simulink model "testemplanner_cs"  (R2023a)
settings: Solver=ode5  StartTime=0.0  StopTime=70  FixedStep=1/1000  RelTol=1e-3
PreLoadFcn:
  | mbxruntime.callbacks.PreLoadFcn(bdroot);
PostLoadFcn:
  | mbxruntime.callbacks.PostLoadFcn(bdroot);
InitFcn:
  | mbxruntime.callbacks.InitFcn(bdroot);
StartFcn:
  | mbxruntime.callbacks.StartFcn(bdroot);
StopFcn:
  | mbxruntime.callbacks.StopFcn(bdroot);
model workspace (MAT data in the model file):
  mbox_table : object (value not decoded)
  model_closed = 0
  sim_status = 0
values from neighbouring files (symbols this model uses):
  c_factor = 43.75    [emplanner_init.m]
  cf = -175016    [emplanner_init.m]
  cr = -130634    [emplanner_init.m]
  global_path_x = [-4.4795 -3.48011774493 -2.48199463442 -1.48514775065 -0.489582877207 0.504698358082 1.49769585569 2.48941007764 3.47984169183 4.46899144113 5.45686009523 6.44344843293 ... (3001 elements, 3001x1)]    [global_path.mat]
  global_path_y = [6.0531 6.0531 6.0531 6.0531 6.0531 6.0531 6.0531 6.0531 6.0531 6.0531 6.0531 6.0531 ... (3001 elements, 3001x1)]    [global_path.mat]
  KD_PID_distance = 0.0    (= 0)    [emplanner_init.m]
  KD_PID_speed = 0    [emplanner_init.m]
  KI_PID_distance = 0.0    (= 0)    [emplanner_init.m]
  KI_PID_speed = 0    [emplanner_init.m]
  KP_PID_distance = 0.5    [emplanner_init.m]
  KP_PID_speed = 1.8    [emplanner_init.m]
  la = 1.265    [emplanner_init.m]
  lb = 2.947-1.265    (= 1.682)    [emplanner_init.m]
  LQR_K1 = k(:,1)'    [emplanner_init.m]
  LQR_K2 = k(:,2)'    [emplanner_init.m]
  LQR_K3 = k(:,3)'    [emplanner_init.m]
  LQR_K4 = k(:,4)'    [emplanner_init.m]
  m = 2020    [emplanner_init.m]
  rack_displacement = [-39.14 , -37.2 , -35.29 , -33.43 , -31.6 , -29.81 , -28.06 , -26.34 , -24.66 ,      -23.01 , -21.38 , -19.79 , -18.23 , -16.69 , -15.18 , -13.7 , -12.23 , -10.8 , -9.38 , -7.98 ,     -6.61 , -5.25 , -3.91 , -2.59 , -1.29 , 0 , 1.27 , 2.54 , 3.78 , 5.02 , 6.24 , 7.46 , 8.66 ,      9.86 , 11.05 , 12.24 , 13.41 , 14.59 , 15.76 , 16.92 , 18.09 , 19.25 , 20.42 , 21.59 , 22.76 ,      23.93 , 25.11 , 26 ...(+26 chars)    [emplanner_init.m]
  right_wheel_ground = [-70 ,-67.2 , -64.4 , -61.6 , -58.8 , -56 , -53.2 , -50.4 , -47.6 , -44.8 , -42 ,      -39.2 , -36.4 , -33.6 , -30.8 , -28 , -25.2 , -22.4 , -19.6 , -16.8 , -14 , -11.2 , -8.4 , -5.6 ,      -2.8 , 0 , 2.8 , 5.6 , 8.4 , 11.2 , 14 , 16.8 , 19.6 , 22.4 , 25.2 , 28 , 30.8 , 33.6 , 36.4 ,      39.2 , 42 , 44.8 , 47.6 , 50.4 , 53.2 , 56 , 58.8 , 61.6 , 64.4 , 67.2 , 70 ]    [emplanner_init.m]
  vx_break_point = zeros(1,5000)    [emplanner_init.m]
undefined symbols (not defined in the file or in its folder): aubr, DiscIntNeverNeededParam, tablebr, vubr, warningInitialVelocity, x0
libraries: PreScanSimulinkLibrary x19, simulink x19, simulink_extras x6, Solver_SF x1
(part 9 of 10)

== matlab function testemplanner_cs/Audi_A8_Sedan_1/decision&planning module/EM Planner/Dynamic Programming ==
  data: dp_path_s output; dp_path_l output; planning_start_s input; planning_start_l input; planning_start_dl input; planning_start_ddl input; obs_s_set input; obs_l_set input; row input; col input; sample_s input; sample_l input; w_dl_smooth_cost input; w_ddl_smooth_cost input; w_dddl_smooth_cost input; w_reference_cost input; w_collision_cost input
function [dp_path_s, dp_path_l] = fcn(planning_start_s, planning_start_l, planning_start_dl, planning_start_ddl, obs_s_set,...
    obs_l_set, row, col, sample_s, sample_l, w_dl_smooth_cost, w_ddl_smooth_cost, w_dddl_smooth_cost, w_reference_cost, w_collision_cost)

%该函数是动态规划（决策算法）的主函数
%要写的太多了，想起什么写什么吧

%node_cost(i,j)为起点到当前节点的最小代价
%每一列中有一个最小的数，代表起点到该列的最小代价
%最后一列的最小数即为起点到最后一列的最小代价，即为我们需要的粗解

%初始化
node_cost = ones(row, col)*inf;
point_s = zeros(row,col);
point_l = zeros(row, col);
point_dl = zeros(row, col);
point_ddl = zeros(row, col);

%下面会计算起点到第一列的最小代价
for i = 1:row
    point_s(i, 1) = planning_start_s+sample_s;
    %对于某奇数行的点阵，例如row=3,point_l(11)=1*sample_l,point_l(31)=-1*sample_l
    point_l(i, 1) = ((row+1)/2-i)*sample_l;
    %用五次多项式连接起点到刚刚生成的点
    %五次多项式有六个边界条件
    start_l = planning_start_l;
    start_dl = planning_start_dl;
    start_ddl = 0;
    end_l = ((row+1)/2-i)*sample_l;
    end_dl = 0;
    end_ddl = 0;
    start_s = planning_start_s;
    end_s = planning_start_s+sample_s;
    %下面定义根据起点中点的六个边界条件计算五次多项式
    cofficient = CalcPathFiveCoff(start_s, end_s, start_l, start_dl, start_ddl, end_l, end_dl, end_ddl);

    %已经将起点和第一列的第一个点用五次多项式连接起来，将六个系数提取出来
    a0 = cofficient(1);
    a1 = cofficient(2);
    a2 = cofficient(3);
    a3 = cofficient(4);
    a4 = cofficient(5);
    a5 = cofficient(6);

    %在曲线上均匀提取十个采样点
    sample_point_s = zeros(10,1);
    sample_point_l = zeros(10,1);
    sample_point_dl = zeros(10,1);
    sample_point_ddl = zeros(10,1);
    sample_point_dddl = zeros(10,1);
    for j = 1:10
        sample_point_s(j) = start_s+j*sample_s/10; %（第一个）采样点的s
    end

    %五次多项式为：a0+a1*s+a2*s^2+a3*s^3+a4*s^4+a5*s^5,根据采样点s计算l,dl,ddl,dddl
    sample_point_l = a0+a1*sample_point_s+a2*sample_point_s.^2+a3*sample_point_s.^3+a4*sample_point_s.^4+...
        a5*sample_point_s.^5;
    sample_point_dl = a1+2*a2*sample_point_s+3*a3*sample_point_s.^2+4*a4*sample_point_s.^3+5*a5*sample_point_s.^4;
    sample_point_ddl = 2*a2+6*a3*sample_point_s+12*a4*sample_point_s.^2+20*a5*sample_point_s.^3;
    sample_point_dddl = 6*a3+24*a4*sample_point_s+60*a5*sample_point_s.^2;
    
    %计算平滑代价、参考线距离代价
    smooth_cost = w_dl_smooth_cost*(sample_point_dl'*sample_point_dl)+w_ddl_smooth_cost*(sample_point_ddl'*sample_point_ddl)...
        +w_dddl_smooth_cost*(sample_point_dddl'*sample_point_dddl);
    reference_cost = w_reference_cost*(sample_point_l'*sample_point_l);

    %定义障碍物代价函数,遍历每个障碍物计算代价做累加
    collision_cost = 0;
    for k = 1:length(obs_s_set)
        if isnan(obs_s_set(k))
            break;
        end
        collision_cost_once = CalcCollCost(sample_point_s, sample_point_l, obs_s_set(k), obs_l_set(k), w_collision_cost);
        collision_cost = collision_cost+collision_cost_once; 
    end

    %计算第一列每个点到起点的node_cost
    node_cost(i, 1) = smooth_cost+reference_cost+collision_cost;

end

%下面将计算从第二列开始每一个点的node_cost
%定义pre_node_index，用来记录当前点的最优路径下，上一个点所对应的行号（列号为当前点-1，无需记录）
%例如有如下点阵,最优路径为（33）<（22）<(11)
%...
%...
%...
%则pre_node_index(33)=2,pre_node_index(22)=1,pre_node_index(11)=0(行数0表示起点)

%初始化pre_node_index矩阵，其值均设为0
pre_node_index = zeros(row, col);

%下面是动态规划的主函数(从第二列开始)
for j = 2:col
    for i = 1:row
        %例如node_cost(1,j)=node_cost(i,j-1)+neighbor_cost(i,j-1)>(1,j)
        %下面要写遍历算法，记录下第二列每个点的node_cost（遍历的是第一列每个点的代价）及pre_node_index
        current_point_s = planning_start_s+j*sample_s;
        current_point_l = ((row+1)/2-i)*sample_l;
        for k = 1:row
            %调用计算相邻点代价的函数
            start_point_s = planning_start_s+(j-1)*sample_s;
            start_point_l = ((row+1)/2-k)*sample_l;
            neighbor_cost = CalcNeighborCost(start_point_s, start_point_l, w_dl_smooth_cost...
            , w_ddl_smooth_cost, w_dddl_smooth_cost, sample_s, obs_s_set, current_point_s, ...
            current_point_l);
            temp_node_cost = node_cost(k, j-1)+neighbor_cost;
            if temp_node_cost < node_cost(i, j)
                node_cost(i, j) = temp_node_cost;
                pre_node_index(i, j) = k;
            end

        end
    end
end

%到这里就写完了动态规划的大部分内容，可以遍历最后一列得到最小代价，以及此路径对应的上一列的行数
%反向递推到第一列就获得了动态规划的结果（粗解）

%row_line（i)为粗解的第i列所对应的行号
row_line = zeros(col, 1);
min_node_cost = inf;

for i = 1:row
    if node_cost(i, col) < min_node_cost
        min_node_cost = node_cost(i, col);
        row_line(col) = i;
    end
end

%映射最优点的pre_node_index,也就是上一列的行号
for j = col-1:-1:1
    row_line(j) = pre_node_index(row_line(j+1), j+1);
end

%将输出初始化，由于事先不知道横纵向的采样数，因此要做缓冲
dp_path_s = ones(15, 1)*-1;
dp_path_l = ones(15, 1)*-1;
for i = 1:col
    dp_path_s(i) = planning_start_s+i*sample_s;
    dp_path_l(i) = ((row+1)/2-row_line(i))*sample_l;
end

%这里定义计算临近点代价的函数，与第一列到起点代价的计算很接近，注意起始点dl,ddl不同...
    function neighbor_cost = CalcNeighborCost(start_point_s, start_point_l, w_dl_smooth_cost...
            , w_ddl_smooth_cost, w_dddl_smooth_cost, sample_s, obs_s_set, current_point_s, ...
            current_point_l)

        %用五次多项式连接起点到刚刚生成的点
        %五次多项式有六个边界条件
        start_l = start_point_l;
        start_dl = 0;
        start_ddl = 0;
        end_l = current_point_l;
        end_dl = 0;
        end_ddl = 0;
        start_s = start_point_s;
        end_s = current_point_s;
        %下面定义根据起点中点的六个边界条件计算五次多项式
        cofficient = CalcPathFiveCoff(start_s, end_s, start_l, start_dl, start_ddl, end_l, end_dl, end_ddl);
    
        %已经将起点和第一列的第一个点用五次多项式连接起来，将六个系数提取出来
        a0 = cofficient(1);
        a1 = cofficient(2);
        a2 = cofficient(3);
        a3 = cofficient(4);
        a4 = cofficient(5);
        a5 = cofficient(6);
    
        %在曲线上均匀提取十个采样点
        sample_point_s = zeros(10,1);
        sample_point_l = zeros(10,1);
        sample_point_dl = zeros(10,1);
        sample_point_ddl = zeros(10,1);
        sample_point_dddl = zeros(10,1);
        for m = 1:10
            sample_point_s(m) = start_s+m*sample_s/10; %（第一个）采样点的s
        end
    
        %五次多项式为：a0+a1*s+a2*s^2+a3*s^3+a4*s^4+a5*s^5,根据采样点s计算l,dl,ddl,dddl
        sample_point_l = a0+a1*sample_point_s+a2*sample_point_s.^2+a3*sample_point_s.^3+a4*sample_point_s.^4+...
            a5*sample_point_s.^5;
        sample_point_dl = a1+2*a2*sample_point_s+3*a3*sample_point_s.^2+4*a4*sample_point_s.^3+5*a5*sample_point_s.^4;
        sample_point_ddl = 2*a2+6*a3*sample_point_s+12*a4*sample_point_s.^2+20*a5*sample_point_s.^3;
        sample_point_dddl = 6*a3+24*a4*sample_point_s+60*a5*sample_point_s.^2;
        
        %计算平滑代价、参考线距离代价
        smooth_cost = w_dl_smooth_cost*(sample_point_dl'*sample_point_dl)+w_ddl_smooth_cost*(sample_point_ddl'*sample_point_ddl)...
            +w_dddl_smooth_cost*(sample_point_dddl'*sample_point_dddl);
        reference_cost = w_reference_cost*(sample_point_l'*sample_point_l);
    
        %定义障碍物代价函数,遍历每个障碍物计算代价做累加
        collision_cost = 0;
        for n = 1:length(obs_s_set)
            if isnan(obs_s_set(n))
                break;
            end
            collision_cost_once = CalcCollCost(sample_point_s, sample_point_l, obs_s_set(n), obs_l_set(n), w_collision_cost);
            collision_cost = collision_cost+collision_cost_once; 
        end
    
        %计算相邻两点的neighbor_cost
        neighbor_cost = smooth_cost+reference_cost+collision_cost;

    end

%在这里定义碰撞代价函数
    function collision_cost = CalcCollCost(sample_point_s, sample_point_l, obs_s, obs_l, w_collision_cost)

        collision_cost = 0; 
        %我们认为障碍物与自车距离大于4米时无代价，3<距离<4时代价为1000/square_distance,距离<3时代价为w_collision_cost
        %其中square_distance为ds^2+dl^2,也就是距离的平方
        ds = (obs_s*ones(10,1)-sample_point_s);
        dl = (obs_l*ones(10,1)-sample_point_l);
        square_distance = ds.^2+dl.^2;
        for q = 1:length(square_distance)
            if square_distance(q) > 9 && square_distance(q) < 16
                collision_cost = collision_cost+1000/square_distance(q);
            elseif square_distance(q) < 9
                collision_cost = collision_cost+w_collision_cost;        
            end
        end
    end

%在这里定义计算五次多项式的函数
function Path_Five_Coff = CalcPathFiveCoff(start_s, end_s, start_l, start_dl, start_ddl, end_l, end_dl, end_ddl)
    %l = a0+a1*s+a2*s^2+a3*s^3+a4*s^4+a5*s^5
    %dl = a1+2*a2*s+3*a3*s^2+4*a4*s^3+5*a5*s^4
    %ddl = 2*a2+6*a3*s+12*a4*s^2+20*a5*s^3
    
    A = [1, start_s, start_s^2, start_s^3, start_s^4, start_s^5;
         0, 1, 2*start_s, 3*start_s^2, 4*start_s^3, 5*start_s^4;
         0, 0, 2, 6*start_s, 12*start_s^2, 20*start_s^3;
         1, end_s, end_s^2, end_s^3, end_s^4, end_s^5;
         0, 1, 2*end_s, 3*end_s^2, 4*end_s^3, 5*end_s^4;
         0, 0, 2, 6*end_s, 12*end_s^2, 20*end_s^3];

    B = [start_l;
         start_dl;
         start_ddl;
         end_l;
         end_dl;
         end_ddl];

    Path_Five_Coff = A\B;
end
end

== matlab function testemplanner_cs/Audi_A8_Sedan_1/decision&planning module/EM Planner/MATLAB Function ==
  data: dp_path_s_init input; dp_path_s_final output; dp_path_l_init input; plan_start_s input; plan_start_l input; plan_start_dl input; plan_start_ddl input; dp_path_l_final output; dp_path_dl_final output; dp_path_ddl_final output
function [dp_path_s_final, dp_path_l_final, dp_path_dl_final, dp_path_ddl_final] = fcn(dp_path_s_init, dp_path_l_init, plan_start_s, plan_start_l...
    , plan_start_dl, plan_start_ddl)

%dp_path_x_init中s方向每隔10m采样一个点，并不是一条密集连续的轨迹，要对轨迹增密
%我们并不知道s方向的采样间隔是多少（可能是10，12，15...），但传感器能探测到的范围大概为60m
%假设ds=1，即每隔1m采样一个点，设置最终轨迹的大小为60，即最多存储60个点（设置缓冲）

ds = 1;
dp_path_s_final = ones(60, 1)*nan;
dp_path_l_final = ones(60, 1)*nan;
dp_path_dl_final = ones(60, 1)*nan;
dp_path_ddl_final = ones(60, 1)*nan;

%设置动态数组用来存储采样点
l_temp = [];
dl_temp = [];
ddl_temp = [];

%设置五次多项式起点
start_s = plan_start_s;
start_l = plan_start_l;
start_dl = plan_start_dl;
start_ddl = plan_start_ddl;

for i = 1:length(dp_path_s_init)
    
    %声明一个动态数组存放采样点的s
    s_cur = [];

    if dp_path_s_init(i) == -1
        break;
    end
    
    %设置内层循环，终点是final_path_s_init(i)
    for j = 1:10000
        s_node = start_s+(j-1)*ds;
        if s_node < dp_path_s_init(i)
            s_cur = [s_cur, s_node];
        else
            break;
        end
    end

    %设置五次多项式终点
    end_s = dp_path_s_init(i);
    end_l = dp_path_l_init(i);
    end_dl = 0;
    end_ddl = 0;
    
    %调用五次多项式函数求解s_cur所对应的l
    Coff = CalcPathFiveCoff(start_s, end_s, start_l, start_dl, start_ddl, end_l, end_dl, end_ddl);
    a0 = Coff(1);
    a1 = Coff(2);
    a2 = Coff(3);
    a3 = Coff(4);
    a4 = Coff(5);
    a5 = Coff(6);
    l = a0*ones(1, length(s_cur))+a1*s_cur+a2*s_cur.^2+a3*s_cur.^3+a4*s_cur.^4+a5*s_cur.^5;
    dl = a1*ones(1, length(s_cur))+2*a2*s_cur+3*a3*s_cur.^2+4*a4*s_cur.^3+5*a5*s_cur.^4;
    ddl = 2*a2*ones(1, length(s_cur))+6*a3*s_cur+12*a4*s_cur.^2+20*a5*s_cur.^3;
    l_temp = [l_temp, l];
    dl_temp = [dl_temp, dl];
    ddl_temp = [ddl_temp, ddl];

    %给s,lfinal赋值，注意l,dl,ddl是扩展的，s_cur是一次性的，每次循环最后要清零
    for k = 1:length(l_temp)
        if k == 61
            break;
        end
        dp_path_s_final(k) = plan_start_s+(k-1)*ds;
        dp_path_l_final(k) = l_temp(k);
        dp_path_dl_final(k) = dl_temp(k);
        dp_path_ddl_final(k) = ddl_temp(k);
    end
 
    %为下一次循环赋值
    start_s = end_s;
    start_l = end_l;
    start_dl = end_dl;
    start_ddl = end_ddl;
   
end

end

%在这里定义计算五次多项式的函数
function Path_Five_Coff = CalcPathFiveCoff(start_s, end_s, start_l, start_dl, start_ddl, end_l, end_dl, end_ddl)
    %l = a0+a1*s+a2*s^2+a3*s^3+a4*s^4+a5*s^5
    %dl = a1+2*a2*s+3*a3*s^2+4*a4*s^3+5*a5*s^4
    %ddl = 2*a2+6*a3*s+12*a4*s^2+20*a5*s^3
    
    A = [1, start_s, start_s^2, start_s^3, start_s^4, start_s^5;
         0, 1, 2*start_s, 3*start_s^2, 4*start_s^3, 5*start_s^4;
         0, 0, 2, 6*start_s, 12*start_s^2, 20*start_s^3;
         1, end_s, end_s^2, end_s^3, end_s^4, end_s^5;
         0, 1, 2*end_s, 3*end_s^2, 4*end_s^3, 5*end_s^4;
         0, 0, 2, 6*end_s, 12*end_s^2, 20*end_s^3];

    B = [start_l;
         start_dl;
         start_ddl;
         end_l;
         end_dl;
         end_ddl];

    Path_Five_Coff = A\B;
end

== matlab function testemplanner_cs/Audi_A8_Sedan_1/decision&planning module/EM Planner/Frenet2Cartesian ==
  data: s_set input; l_set input; dl_set input; ddl_set input; frenet_x input; frenet_y input; frenet_heading input; frenet_kappa input; index2s input; x_point_set output; y_point_set output; heading_point_set output; kappa_point_set output
function [x_point_set, y_point_set, heading_point_set, kappa_point_set] = fcn(s_set, l_set, dl_set, ddl_set, frenet_x, ...
    frenet_y, frenet_heading, frenet_kappa, index2s)

%该函数的作用是把自然坐标系(s,l)下的粗解转换到笛卡尔坐标系（x,y）
%不确定有多少个点需要坐标转换，要做缓冲
%frenet转cartesian的步骤是：先找到待变换点在参考线上投影点的x,y，再计算待转换点的x,y

%在index2s上遍历得到匹配点编号，用匹配点求投影点的xy...

%这里可能有bug,因为s是点的投影的弧长，而不是点的匹配点的弧长，我认为找到在参考线上索引之后可以直接得到投影点的几何信息

x_point_set = ones(128, 1)*nan;
y_point_set = ones(128, 1)*nan;
heading_point_set = ones(128, 1)*nan;
kappa_point_set = ones(128, 1)*nan; 

for i = 1:length(s_set)
    if isnan(s_set(i))
        break;
    end
    %调用函数计算投影点
    [proj_point, proj_point_x, proj_point_y, proj_point_heading, proj_point_kappa] = CalcProjPoint(index2s, s_set(i), frenet_x, frenet_y, frenet_heading, frenet_kappa);
    %根据投影点的xy计算待转换点的xy
    proj_nor = [-sin(proj_point_heading); cos(proj_point_heading)];
    point = proj_point+proj_nor*l_set(i);
    x_point_set(i) = point(1);
    y_point_set(i) = point(2);
    heading_point_set(i) = atan(dl_set(i)/(1-proj_point_kappa*l_set(i)))+proj_point_heading;
    %近似认为kr'=0
    kappa_point_set(i) = ((ddl_set(i)+proj_point_kappa*dl_set(i)*tan(heading_point_set(i)-proj_point_heading))...
        *(cos(heading_point_set(i)-proj_point_heading)^2)/(1-proj_point_kappa*l_set(i))+proj_point_kappa)*cos(heading_point_set(i)-proj_point_heading)...
        /(1-proj_point_kappa*l_set(i));

end

end

%定义计算投影点的函数
function [proj_point, proj_point_x, proj_point_y, proj_point_heading, proj_point_kappa] = CalcProjPoint(index2s, s, frenet_x, frenet_y, frenet_heading, frenet_kappa)

%先遍历找到index2s上的匹配点
match_index = 1;
while index2s(match_index) < s
    match_index = match_index+1;
end
%提取数据（按照上述做法，匹配点一定在投影点之后，感觉有bug）
match_point = [frenet_x(match_index); frenet_y(match_index)];
match_point_heading = frenet_heading(match_index);
match_point_kappa = frenet_kappa(match_index);
ds = s-index2s(match_index);
match_tor = [cos(match_point_heading); sin(match_point_heading)];
proj_point = match_point+ds*match_tor;
proj_point_x = proj_point(1);
proj_point_y = proj_point(2);
proj_point_heading = match_point_heading+ds*match_point_kappa;
proj_point_kappa = match_point_kappa;
end

== matlab function testemplanner_cs/Audi_A8_Sedan_1/decision&planning module/referenceline provider/match&proj point search1 ==
  data: match_point_index_set output; proj_x_set output; proj_y_set output; proj_heading_set output; proj_kappa_set output; x_set input; y_set input; frenet_x_set input; frenet_y_set input; frenet_heading_set input; frenet_kapppa_set input
function [match_point_index_set, proj_x_set, proj_y_set, proj_heading_set, proj_kappa_set] = fcn(x_set, y_set, frenet_x_set, frenet_y_set, ...
    frenet_heading_set, frenet_kapppa_set)

%待投影点是一个集合（自车，障碍物），每一个点分别遍历寻找匹配点，再寻找投影点
%匹配点集合要保存下来，作为下次遍历开始的起点
%第一次遍历，没有任何提示，从frenet点集第一点开始遍历
%若不是第一次遍历，从上次保存的匹配点开始，注意方向
%待投影点-寻找匹配点-寻找投影点-投影点（x,y,heading,kappa），保存匹配点索引集合

%（待）投影点数量未知，设置缓冲，最多批量处理128个点,信息冗余用NAN（not a number）处理
n = 128;
match_point_index_set = ones(n,1)*nan;
proj_x_set = ones(n,1)*nan;
proj_y_set = ones(n,1)*nan;
proj_heading_set = ones(n,1)*nan;
proj_kappa_set = ones(n,1)*nan;

%两种情况：第一次遍历，非第一次遍历
%声明两个全局变量，第一个用来判断是否初次运行，第二个用来存储上次匹配点集合
persistent is_first_run
persistent pre_match_point_index_set

if isempty(is_first_run)
    is_first_run = 0;
    pre_match_point_index_set = ones(n,1)*nan;
    %遍历每一个点寻找匹配点
    start_search_index = 1;
    for i = 1:length(x_set)
        if isnan(x_set(i))
            break;
        end
        increase_count = 0;
        min_distant = inf;
        for j = start_search_index:length(frenet_x_set)
            distant = (x_set(i)-frenet_x_set(j))^2+(y_set(i)-frenet_y_set(j))^2;
            if distant < min_distant
                min_distant = distant;
                increase_count = 0;
                match_point_index_set(i) = j;
            else
                increase_count = increase_count+1;
            end
            %第一次遍历连续增加50次停止
            if increase_count > 50
                break;
            end
        end
        %通过匹配点计算投影点
        %计算匹配点的位矢及方向向量
        vector_match_point = [frenet_x_set(match_point_index_set(i));frenet_y_set(match_point_index_set(i))];
        vector_match_point_direction = [cos(frenet_heading_set(match_point_index_set(i)));sin(frenet_heading_set(match_point_index_set(i)))];
        vector_d = [x_set(i);y_set(i)]-vector_match_point;
        ds = vector_d'*vector_match_point_direction;
        vector_ds = ds*vector_match_point_direction;
        vector_proj_point = vector_match_point+vector_ds;
        %计算投影点的x,y,heading,kappa
        proj_x_set(i) = vector_proj_point(1);
        proj_y_set(i) = vector_proj_point(2);
        proj_heading_set(i) = frenet_heading_set(match_point_index_set(i))+frenet_kapppa_set(match_point_index_set(i))*ds;
        proj_kappa_set(i) = frenet_kapppa_set(match_point_index_set(i));
    end
    pre_match_point_index_set = match_point_index_set;
else
    %如果不是第一次遍历
    for i = 1:length(x_set)

        if isnan(x_set(i))
            break;
        end
        %下面这行代码有严重问题，需要投影的不仅是自车，还有障碍物
        %而第一次运行时传感器可能监测不到障碍物，即算法会跳过is first run分支执行else分支
        %此时pre_match_point_index_set中除了自车都是nan，所以需要修复
        start_search_index = pre_match_point_index_set(i);
        increase_count_limit = 5;

        if isnan(start_search_index)
            %从第一个点开始遍历，并需要遍历50次防止取到局部极小值
            increase_count_limit = 50;
            start_search_index = 1;
        end

        increase_count = 0;
        min_distant = inf;
        %判断遍历方向
        vector_pre_match_point = [frenet_x_set(start_search_index);frenet_y_set(start_search_index)];
        vector_pre_match_point_direction = [cos(frenet_heading_set(start_search_index));sin(frenet_heading_set(start_search_index))];
        flag = ([x_set(i);y_set(i)]-vector_pre_match_point)'*vector_pre_match_point_direction;
        

        %正向遍历
        if flag > 0.001
            for j = start_search_index:length(frenet_x_set)
                distant = (x_set(i)-frenet_x_set(j))^2+(y_set(i)-frenet_y_set(j))^2;
                if distant < min_distant
                    min_distant = distant;
                    increase_count = 0;
                    match_point_index_set(i) = j;
                else
                    increase_count = increase_count+1;
                end
                %连续增加5次停止
                if increase_count > increase_count_limit
                    break;
                end
            end
            % %通过匹配点计算投影点
            % %计算匹配点的位矢及方向向量
            % vector_match_point = [frenet_x_set(match_point_index_set(i));frenet_y_set(match_point_index_set(i))];
            % vector_match_point_direction = [cos(frenet_heading_set(match_point_index_set(i)));sin(frenet_heading_set(match_point_index_set(i)))];
            % vector_d = [x_set(i);y_set(i)]-vector_match_point;
            % ds = vector_d'*vector_match_point_direction;
            % vector_ds = ds*vector_match_point_direction;
            % vector_proj_point = vector_match_point+vector_ds;
            % %计算投影点的x,y,heading,kappa
            % proj_x_set(i) = vector_proj_point(1);
            % proj_y_set(i) = vector_proj_point(2);
            % proj_heading_set(i) = frenet_heading_set(match_point_index_set(i))+frenet_kapppa_set(match_point_index_set(i))*ds;
            % proj_kappa_set(i) = frenet_kapppa_set(match_point_index_set(i));
        elseif flag < -0.001
            %反向遍历
             for j = start_search_index:-1:1
                distant = (x_set(i)-frenet_x_set(j))^2+(y_set(i)-frenet_y_set(j))^2;
                if distant < min_distant
                    min_distant = distant;
                    increase_count = 0;
                    match_point_index_set(i) = j;
                else
                    increase_count = increase_count+1;
                end
                %连续增加5次停止
                if increase_count > increase_count_limit
                    break;
                end
            end
        else
            match_point_index_set(i) = start_search_index;
        end

        %通过匹配点计算投影点
        %计算匹配点的位矢及方向向量
        vector_match_point = [frenet_x_set(match_point_index_set(i));frenet_y_set(match_point_index_set(i))];
        vector_match_point_direction = [cos(frenet_heading_set(match_point_index_set(i)));sin(frenet_heading_set(match_point_index_set(i)))];
        vector_d = [x_set(i);y_set(i)]-vector_match_point;
        ds = vector_d'*vector_match_point_direction;
        vector_ds = ds*vector_match_point_direction;
        vector_proj_point = vector_match_point+vector_ds;
        %计算投影点的x,y,heading,kappa
        proj_x_set(i) = vector_proj_point(1);
        proj_y_set(i) = vector_proj_point(2);
        proj_heading_set(i) = frenet_heading_set(match_point_index_set(i))+frenet_kapppa_set(match_point_index_set(i))*ds;
        proj_kappa_set(i) = frenet_kapppa_set(match_point_index_set(i));

    end
    pre_match_point_index_set = match_point_index_set;
end

== matlab function testemplanner_cs/Audi_A8_Sedan_1/decision&planning module/EM Planner/calc path length and map between point and s ==
  data: trajectory_x input; path_s_end output; trajectory_y input; path_s output
function [path_s_end,path_s] = fcn(trajectory_x,trajectory_y)
% 该函数将计算以trajectory的s 与 x y 的对应关系，可以看作是trajectory index2s
n = length(trajectory_x);
path_s = zeros(n,1);
sum = 0;
for i = 2:length(trajectory_x)
    if isnan(trajectory_x(i))
        break;
    end
    sum = sum + sqrt((trajectory_x(i) - trajectory_x(i-1))^2 + (trajectory_y(i) - trajectory_y(i-1))^2);
    path_s(i) = sum;
end
% 计算出trajectory的长度
if i == n
    path_s_end = path_s(end);
else
    % 因为循环的退出条件为isnan(trajectory_x(i)) 所以 i 所对应的数为 nan 
    path_s_end = path_s(i - 1);
end

== matlab function testemplanner_cs/Audi_A8_Sedan_1/decision&planning module/EM Planner/increase st point count ==
  data: s_init input; s output; s_dot_init input; s_dot2_init input; relative_time_init input; s_dot output; s_dot2 output; relative_time output
function [s,s_dot,s_dot2,relative_time] = fcn(s_init,s_dot_init,s_dot2_init,relative_time_init)
%该函数将增密s s_dot s_dot2
% 为什么需要增密，因为控制的执行频率是规划的10倍，轨迹点如果不够密，必然会导致规划效果不好
% 但是若在速度二次规划中点取的太多，会导致二次规划的矩阵规模太大计算太慢
% 所以方法是在二次规划中选取少量的点优化完毕后，在用此函数增密
T = relative_time_init(end);
n = 401;
dt = T/(n-1);
s = zeros(n,1);
s_dot = zeros(n,1);
s_dot2 = zeros(n,1);
relative_time = zeros(n,1);
for i = 1:n
    current_t = (i-1)*dt;
    for j = 1:length(relative_time_init)-1
        if relative_time_init(j) <= current_t && relative_time_init(j+1) > current_t
            break;
        end
    end
    x = current_t - relative_time_init(j);
    s(i) = s_init(j) + s_dot_init(j)*x + (1/3)*s_dot2_init(j)*x^2 + (1/6)*s_dot2_init(j+1)*x^2; 
    s_dot(i) = s_dot_init(j) + 0.5*s_dot2_init(j)*x + 0.5*s_dot2_init(j+1)*x;
    s_dot2(i) = s_dot2_init(j) + (s_dot2_init(j+1) - s_dot2_init(j))*x/(relative_time_init(j+1) - relative_time_init(j));
    relative_time(i) = current_t;
end

== matlab function testemplanner_cs/Audi_A8_Sedan_1/decision&planning module/EM Planner/path and speed merge ==
  data: s input; trajectory_x output; s_dot input; s_dot2 input; relative_time input; current_time input; path_s input; trajectory_x_init input; trajectory_y_init input; trajectory_heading_init input; trajectory_kappa_init input; trajectory_y output; trajectory_heading output; trajectory_kappa output; trajectory_speed output; trajectory_accel output; trajectory_time output
function [trajectory_x,trajectory_y,trajectory_heading,trajectory_kappa,trajectory_speed,trajectory_accel,trajectory_time] = ...
    fcn(s,s_dot,s_dot2,relative_time,current_time,path_s,trajectory_x_init,trajectory_y_init,trajectory_heading_init,trajectory_kappa_init)
% 该函数将合并path和speed
% 由于path 是 60个点，speed 有 401个点，合并后，path和speed有401个点，因此需要做插值
n = 401;
trajectory_x = zeros(n,1);
trajectory_y = zeros(n,1);
trajectory_heading = zeros(n,1);
trajectory_kappa = zeros(n,1);
trajectory_speed = zeros(n,1);

trajectory_accel = zeros(n,1);
index = 1;
% 由于trajectory_x_init中不是所有的值都有效，(有nan) 所以要找到有效值的范围
while ~isnan(trajectory_x_init(index)) 
    index = index + 1;
end
index = index - 1;
trajectory_time = zeros(n,1);
for i = 1:n-1
    %interp1 线性插值
    % 若 x = [1,2] y = [3,4]
    %interp1(x,y,1.5) 会得到3.5
    %interp1 的缺点是 在端点或超过端点的，结果为nan
    % interp1(x,y,2) 不会等于4 而是会等于nan
    % interp1(x,y,6) 也会等于nan，所以在端点处要单独处理
    trajectory_x(i) = interp1(path_s(1:index),trajectory_x_init(1:index),s(i));
    trajectory_y(i) = interp1(path_s(1:index),trajectory_y_init(1:index),s(i));
    trajectory_heading(i) = interp1(path_s(1:index),trajectory_heading_init(1:index),s(i));
    trajectory_kappa(i) = interp1(path_s(1:index),trajectory_kappa_init(1:index),s(i));
    trajectory_time(i) = relative_time(i) + current_time;%速度规划会得到相对时间，转换成绝对时间
    trajectory_speed(i) = s_dot(i);
    trajectory_accel(i) = s_dot2(i);
end
% 端点单独处理
trajectory_x(end) = trajectory_x_init(end);
trajectory_y(end) = trajectory_y_init(end);
trajectory_heading(end) = trajectory_heading_init(end);
trajectory_kappa(end) = trajectory_kappa_init(end);
trajectory_time(end) = relative_time(end) + current_time;
trajectory_speed(end) = s_dot(end);
trajectory_accel(end) = s_dot2(end);

== matlab function testemplanner_cs/Audi_A8_Sedan_1/decision&planning module/EM Planner/stitch trajectory ==
  data: trajectory_x input; trajectory_x_final output; trajectory_y input; trajectory_heading input; trajectory_kappa input; trajectory_speed input; trajectory_accel input; trajectory_time input; stitch_x input; stitch_y input; stitch_heading input; stitch_kappa input; stitch_speed input; stitch_accel input; stitch_time input; trajectory_y_final output; trajectory_heading_final output; trajectory_kappa_final output; trajectory_speed_final output; trajectory_accel_final output; trajectory_time_final output
function [trajectory_x_final,trajectory_y_final,trajectory_heading_final,trajectory_kappa_final,...
          trajectory_speed_final,trajectory_accel_final,trajectory_time_final] = fcn(trajectory_x,...
          trajectory_y,trajectory_heading,trajectory_kappa,trajectory_speed,trajectory_accel,trajectory_time,...
          stitch_x,stitch_y,stitch_heading,stitch_kappa,stitch_speed,stitch_accel,stitch_time)
% 轨迹拼接，把stitch trajectory 拼到规划完成的轨迹上
n = 401 + 20;
trajectory_x_final = zeros(n,1);
trajectory_y_final = zeros(n,1);
trajectory_heading_final = zeros(n,1);
trajectory_kappa_final = zeros(n,1);
trajectory_speed_final = zeros(n,1);
trajectory_accel_final = zeros(n,1);
trajectory_time_final = zeros(n,1);

trajectory_x_final = [stitch_x;trajectory_x];
trajectory_y_final = [stitch_y;trajectory_y];
trajectory_heading_final = [stitch_heading;trajectory_heading];
trajectory_kappa_final = [stitch_kappa;trajectory_kappa];
trajectory_speed_final = [stitch_speed;trajectory_speed];
trajectory_accel_final = [stitch_accel;trajectory_accel];
trajectory_time_final = [stitch_time;trajectory_time];

== matlab function testemplanner_cs/Audi_A8_Sedan_1/control module/MATLAB Function ==
  data: current_time input; xr output; trajectory_x input; trajectory_y input; trajectory_heading input; trajectory_kappa input; trajectory_speed input; trajectory_accel input; yr output; thetar output; kappar output; speedr output; accelr output; trajectory_time input
function [xr, yr, thetar, kappar, speedr, accelr] = fcn(current_time, trajectory_x, trajectory_y, trajectory_heading...
    , trajectory_kappa, trajectory_speed, trajectory_accel, trajectory_time)

%因为控制接受的信号不再是一个点，而是一个序列，因此要找出控制时间对应的轨迹信息
%控制也有延迟，因此控制跟踪的点的时间应该是当前时间+10ms

control_time = current_time+0.01;

%由于轨迹是拼接而成的，若无拼接轨迹，stitch_time中的信息应该是-1
%所以要找到时间信息中第一个不是-1的点
index = 1;
while trajectory_time(index) == -1
    index = index+1;
end

%用inerp1对时间插值，simulink中该函数要求自变量是线性变化的，且插值时间应该在插值范围之内
%若待插点处在范围边界或之外，会发生报错
%规划的周期是100ms,意味着第一次规划还未完成控制已经执行了十次
%控制跟踪的是一条空轨迹：0,0,0,0,0...,trajectory_time也全部为0(非线性)
%上述情况只可能发生在仿真刚开始时
if control_time > trajectory_time(index) && trajectory_time(index) ~= 0
    xr = interp1(trajectory_time(index:end), trajectory_x(index:end), control_time);
    yr = interp1(trajectory_time(index:end), trajectory_y(index:end), control_time);
    thetar = interp1(trajectory_time(index:end), trajectory_heading(index:end), control_time);
    kappar = interp1(trajectory_time(index:end), trajectory_kappa(index:end), control_time);
    speedr = interp1(trajectory_time(index:end), trajectory_speed(index:end), control_time);
    accelr = interp1(trajectory_time(index:end), trajectory_accel(index:end), control_time);
else
    xr = trajectory_x(index);
    yr = trajectory_y(index);
    thetar = trajectory_heading(index);
    kappar = trajectory_kappa(index);
    speedr = trajectory_speed(index);
    accelr = trajectory_accel(index);
end

== matlab function testemplanner_cs/Audi_A8_Sedan_1/decision&planning module/referenceline provider/match&proj point search2 ==
  data: match_point_index_set output; proj_x_set output; proj_y_set output; proj_heading_set output; proj_kappa_set output; x_set input; y_set input; frenet_x_set input; frenet_y_set input; frenet_heading_set input; frenet_kapppa_set input
function [match_point_index_set, proj_x_set, proj_y_set, proj_heading_set, proj_kappa_set] = fcn(x_set, y_set, frenet_x_set, frenet_y_set, ...
    frenet_heading_set, frenet_kapppa_set)

%待投影点是一个集合（自车，障碍物），每一个点分别遍历寻找匹配点，再寻找投影点
%匹配点集合要保存下来，作为下次遍历开始的起点
%第一次遍历，没有任何提示，从frenet点集第一点开始遍历
%若不是第一次遍历，从上次保存的匹配点开始，注意方向
%待投影点-寻找匹配点-寻找投影点-投影点（x,y,heading,kappa），保存匹配点索引集合

%（待）投影点数量未知，设置缓冲，最多批量处理128个点,信息冗余用NAN（not a number）处理
n = 128;
match_point_index_set = ones(n,1)*nan;
proj_x_set = ones(n,1)*nan;
proj_y_set = ones(n,1)*nan;
proj_heading_set = ones(n,1)*nan;
proj_kappa_set = ones(n,1)*nan;

%两种情况：第一次遍历，非第一次遍历
%声明两个全局变量，第一个用来判断是否初次运行，第二个用来存储上次匹配点集合
persistent is_first_run
persistent pre_match_point_index_set

if isempty(is_first_run)
    is_first_run = 0;
    pre_match_point_index_set = ones(n,1)*nan;
    %遍历每一个点寻找匹配点
    start_search_index = 1;
    for i = 1:length(x_set)
        if isnan(x_set(i))
            break;
        end
        increase_count = 0;
        min_distant = inf;
        for j = start_search_index:length(frenet_x_set)
            distant = (x_set(i)-frenet_x_set(j))^2+(y_set(i)-frenet_y_set(j))^2;
            if distant < min_distant
                min_distant = distant;
                increase_count = 0;
                match_point_index_set(i) = j;
            else
                increase_count = increase_count+1;
            end
            %第一次遍历连续增加50次停止
            if increase_count > 50
                break;
            end
        end
        %通过匹配点计算投影点
        %计算匹配点的位矢及方向向量
        vector_match_point = [frenet_x_set(match_point_index_set(i));frenet_y_set(match_point_index_set(i))];
        vector_match_point_direction = [cos(frenet_heading_set(match_point_index_set(i)));sin(frenet_heading_set(match_point_index_set(i)))];
        vector_d = [x_set(i);y_set(i)]-vector_match_point;
        ds = vector_d'*vector_match_point_direction;
        vector_ds = ds*vector_match_point_direction;
        vector_proj_point = vector_match_point+vector_ds;
        %计算投影点的x,y,heading,kappa
        proj_x_set(i) = vector_proj_point(1);
        proj_y_set(i) = vector_proj_point(2);
        proj_heading_set(i) = frenet_heading_set(match_point_index_set(i))+frenet_kapppa_set(match_point_index_set(i))*ds;
        proj_kappa_set(i) = frenet_kapppa_set(match_point_index_set(i));
    end
    pre_match_point_index_set = match_point_index_set;
else
    %如果不是第一次遍历
    for i = 1:length(x_set)

        if isnan(x_set(i))
            break;
        end
        %下面这行代码有严重问题，需要投影的不仅是自车，还有障碍物
        %而第一次运行时传感器可能监测不到障碍物，即算法会跳过is first run分支执行else分支
        %此时pre_match_point_index_set中除了自车都是nan，所以需要修复
        start_search_index = pre_match_point_index_set(i);
        increase_count_limit = 5;

        if isnan(start_search_index)
            %从第一个点开始遍历，并需要遍历50次防止取到局部极小值
            increase_count_limit = 50;
            start_search_index = 1;
        end

        increase_count = 0;
        min_distant = inf;
        %判断遍历方向
        vector_pre_match_point = [frenet_x_set(start_search_index);frenet_y_set(start_search_index)];
        vector_pre_match_point_direction = [cos(frenet_heading_set(start_search_index));sin(frenet_heading_set(start_search_index))];
        flag = ([x_set(i);y_set(i)]-vector_pre_match_point)'*vector_pre_match_point_direction;
        

        %正向遍历
        if flag > 0.001
            for j = start_search_index:length(frenet_x_set)
                distant = (x_set(i)-frenet_x_set(j))^2+(y_set(i)-frenet_y_set(j))^2;
                if distant < min_distant
                    min_distant = distant;
                    increase_count = 0;
                    match_point_index_set(i) = j;
                else
                    increase_count = increase_count+1;
                end
                %连续增加5次停止
                if increase_count > increase_count_limit
                    break;
                end
            end
            % %通过匹配点计算投影点
            % %计算匹配点的位矢及方向向量
            % vector_match_point = [frenet_x_set(match_point_index_set(i));frenet_y_set(match_point_index_set(i))];
            % vector_match_point_direction = [cos(frenet_heading_set(match_point_index_set(i)));sin(frenet_heading_set(match_point_index_set(i)))];
            % vector_d = [x_set(i);y_set(i)]-vector_match_point;
            % ds = vector_d'*vector_match_point_direction;
            % vector_ds = ds*vector_match_point_direction;
            % vector_proj_point = vector_match_point+vector_ds;
            % %计算投影点的x,y,heading,kappa
            % proj_x_set(i) = vector_proj_point(1);
            % proj_y_set(i) = vector_proj_point(2);
            % proj_heading_set(i) = frenet_heading_set(match_point_index_set(i))+frenet_kapppa_set(match_point_index_set(i))*ds;
            % proj_kappa_set(i) = frenet_kapppa_set(match_point_index_set(i));
        elseif flag < -0.001
            %反向遍历
             for j = start_search_index:-1:1
                distant = (x_set(i)-frenet_x_set(j))^2+(y_set(i)-frenet_y_set(j))^2;
                if distant < min_distant
                    min_distant = distant;
                    increase_count = 0;
                    match_point_index_set(i) = j;
                else
                    increase_count = increase_count+1;
                end
                %连续增加5次停止
                if increase_count > increase_count_limit
                    break;
                end
            end
        else
            match_point_index_set(i) = start_search_index;
        end

        %通过匹配点计算投影点
        %计算匹配点的位矢及方向向量
        vector_match_point = [frenet_x_set(match_point_index_set(i));frenet_y_set(match_point_index_set(i))];
        vector_match_point_direction = [cos(frenet_heading_set(match_point_index_set(i)));sin(frenet_heading_set(match_point_index_set(i)))];
        vector_d = [x_set(i);y_set(i)]-vector_match_point;
        ds = vector_d'*vector_match_point_direction;
        vector_ds = ds*vector_match_point_direction;
        vector_proj_point = vector_match_point+vector_ds;
        %计算投影点的x,y,heading,kappa
        proj_x_set(i) = vector_proj_point(1);
        proj_y_set(i) = vector_proj_point(2);
        proj_heading_set(i) = frenet_heading_set(match_point_index_set(i))+frenet_kapppa_set(match_point_index_set(i))*ds;
        proj_kappa_set(i) = frenet_kapppa_set(match_point_index_set(i));

    end
    pre_match_point_index_set = match_point_index_set;
end

== matlab function testemplanner_cs/Audi_A8_Sedan_1/decision&planning module/EM Planner/path decision with dynamic planning(dp) ==
  data: obs_s_set input; dp_path_s output; obs_l_set input; plan_start_s input; plan_start_l input; plan_start_dl input; plan_start_dll input; w_cost_collision input; w_cost_smooth_dl input; w_cost_smooth_ddl input; w_cost_smooth_dddl input; w_cost_ref input; row input; col input; sample_s input; sample_l input; dp_path_l output
function [dp_path_s,dp_path_l] = fcn(obs_s_set,obs_l_set,plan_start_s,plan_start_l,plan_start_dl,...
    plan_start_dll,w_cost_collision,w_cost_smooth_dl,w_cost_smooth_ddl,w_cost_smooth_dddl,w_cost_ref,row,col,sample_s,sample_l)
%该函数为路径决策算法动态规划的主函数
% 输入：obs s l set 筛选后的障碍物sl信息
%       plan_start s l dl ddl 规划起点信息
%       w_cost_obs,w_cost_smooth_dl,w_cost_smooth_ddl,w_cost_smooth_dddl,w_cost_ref动态规划代价权重
%       row col 动态规划采样点的行数和列数(row必须是奇数，col必须是6)
%       sample_s,sample_l 采样的s l 长度
% 输出：dp_path_l,dp_path_s 动态规划的路径sl,此路径不包含规划起点  

%动态规划最优的数据结构是结构体矩阵，但是simulink不支持结构体矩阵，所以动态规划算法写的相对难以理解

%声明二维矩阵变量node_cost，node_cost(i,j)表示从起点出发，到行i列j节点的最小代价为node_cost(i,j)
node_cost = ones(row,col)*inf;%初始化为无穷大

%声明二维矩阵变量pre_node_index pre_node_index(i,j)表示从起点到行i列j的节点的最优路径中前一个节点的行号为
%pre_node_index(i,j)
%例：比如一条最优路径为 起点 -> node(1,1) -> node(2,2) -> node(3,3)
%则pre_node_index(3,3) = 2 (最优路径的前一个节点是node(2,2) 取它的行号）
%  pre_node_index(2,2) = 1 (最优路径的前一个节点是node(1,1) 取它的行号）
%  pre_node_index(1,1) = 0 (起点的行号默认是0)

% 其实pre_node_index就是当找到最小代价的路径后从终点到起点反向选择出最优路径的
%如果用结构体矩阵完全没有必要弄得这么麻烦，但是simulink不支持
pre_node_index = zeros(row,col);%初始化，所有节点的上个最优节点的行号都是0，也就是起点

%先计算从起点到第一列的cost
for i = 1:row
    node_cost(i,1) = CalcStartCost(plan_start_s,plan_start_l,plan_start_dl,...
    plan_start_dll,i,sample_s,sample_l,w_cost_collision,w_cost_smooth_dl,...
    w_cost_smooth_ddl,w_cost_smooth_dddl,w_cost_ref,obs_s_set,obs_l_set,row);
end
% 动态规划主函数，从第二列开始
for j = 2:col
    for i = 1:row
        %计算当前node(i,j)的s l
        cur_node_s = plan_start_s + j * sample_s;
        cur_node_l = ((row + 1)/2 - i) * sample_l;
        %遍历前一列的节点
        for k = 1:row
            %计算前一列节点的s l
            pre_node_s = plan_start_s + (j - 1) * sample_s;
            pre_node_l = ((row + 1)/2 - k) * sample_l;
            cost_neighbour = CalcNeighbourCost(pre_node_s,pre_node_l,cur_node_s,cur_node_l,w_cost_collision,...
    w_cost_smooth_dl,w_cost_smooth_ddl,w_cost_smooth_dddl,w_cost_ref,obs_s_set,obs_l_set);
            %起点到上一个节点的最小代价为node_cost(k,j-1)
            pre_min_cost = node_cost(k,j-1);
            %起点到node_cost(i,j)的最小代价 为node_cost(k,j-1)
            %再加上node(k,j-1)到node(i,j)的代价 (k = 1,2,3,4...row) 中最小的
            cost_temp = pre_min_cost + cost_neighbour;
            if cost_temp < node_cost(i,j)
                node_cost(i,j) = cost_temp;
                %把最优路径上一列节点的行号记录下来
                pre_node_index(i,j) = k;
            end
        end      
    end
end
%找到node_cost最后一列中，cost最小的，记代价最小的行号为index
index = 0;
min_cost = inf;
for i = 1:row
    if node_cost(i,end) < min_cost
        min_cost = node_cost(i,end);
        index = i;
    end
end
%动态规划最优路径初始化
dp_node_list_row = zeros(col,1);
%从后往前逆推
cur_index = index;
for i = 1:col
    %记录cur_index前面节点的行号
    pre_index = pre_node_index(cur_index,end - i + 1);
    %把cur_index放到dp_node_list_row对应的位置
    dp_node_list_row(col - i + 1) = cur_index;
    %再把pre_index 赋给 cur_index 进行下一步递推
    cur_index = pre_index;
end
% 输出初始化，由于事先不知道横纵向的采样列数，因此需要做缓冲
dp_path_s = ones(15,1)*-1;
dp_path_l = ones(15,1)*-1;
for i = 1:col
    dp_path_s(i) = plan_start_s + i * sample_s;
    dp_path_l(i) = ((row + 1) / 2 - dp_node_list_row(i)) * sample_l;
end








end
function cost = CalcNeighbourCost(pre_node_s,pre_node_l,cur_node_s,cur_node_l,w_cost_collision,...
    w_cost_smooth_dl,w_cost_smooth_ddl,w_cost_smooth_dddl,w_cost_ref,obs_s_set,obs_l_set)
% 该函数将计算相邻两个节点之间的cost
  
    start_l = pre_node_l;
    start_dl = 0;
    start_ddl = 0;
    end_l = cur_node_l;
    end_dl = 0;
    end_ddl = 0;
    start_s = pre_node_s;
    end_s = cur_node_s;
    coeff = CalcQuinticCoeffient(start_l,start_dl,start_ddl,end_l,end_dl,end_ddl,start_s,end_s);
    a0 = coeff(1);
    a1 = coeff(2);
    a2 = coeff(3);
    a3 = coeff(4);
    a4 = coeff(5);
    a5 = coeff(6);
    % 取10个点计算cost
    ds = zeros(10,1);
    l = zeros(10,1);
    dl = zeros(10,1);
    ddl = zeros(10,1);
    dddl = zeros(10,1);
    for i = 1:10
        ds(i) = start_s + (i-1)*(end_s - start_s)/10;
    end
    l = a0 * ones(10,1) + a1 * ds + a2 * ds.^2 + a3 * ds.^3 + a4 * ds.^4 + a5 * ds.^5;
    dl = a1 * ones(10,1) + 2 * a2 * ds + 3 * a3 * ds.^2 + 4 * a4 * ds.^3 + 5 * a5 * ds.^4;
    ddl = 2 * a2 * ones(10,1) + 6 * a3 * ds + 12 * a4 * ds.^2 + 20 * a5 * ds.^3;
    dddl = 6 * ones(10,1) * a3 + 24 * a4 * ds + 60 * a5 * ds.^2;
    cost_smooth = w_cost_smooth_dl * (dl' * dl) + w_cost_smooth_ddl * (ddl' * ddl) + w_cost_smooth_dddl * (dddl' * dddl);
    cost_ref = w_cost_ref * (l' * l);
    cost_collision = 0;
    for i = 1:length(obs_s_set)
        if isnan(obs_s_set(i))
            break;
        end
        dlon = ones(10,1) * obs_s_set(i) - ds;
        dlat = ones(10,1) * obs_l_set(i) - l;
        %这里做了非常简化的质点模型，认为障碍物就是一个点
        square_d = dlon.^2 + dlat.^2;
        cost_collision_once = CalcObsCost(w_cost_collision,square_d);
        cost_collision = cost_collision + cost_collision_once;
    end
    cost = cost_collision + cost_smooth + cost_ref;


end


function cost = CalcStartCost(begin_s,begin_l,begin_dl,begin_ddl,cur_node_row,sample_s,sample_l,w_cost_collision,...
    w_cost_smooth_dl,w_cost_smooth_ddl,w_cost_smooth_dddl,w_cost_ref,obs_s_set,obs_l_set,row)
    %该函数将计算起点到第一层的cost
    start_l = begin_l;
    start_dl = begin_dl;
    start_ddl = begin_ddl;
    %  . . .
    %  . . . row = 3 中间的行号 = (row + 1) /2 = 2
    %  . . .
    end_l = ((row + 1)/2 - cur_node_row)*sample_l;
    end_dl = 0;
    end_ddl = 0;
    start_s = begin_s;
    end_s = begin_s + sample_s;
    coeff = CalcQuinticCoeffient(start_l,start_dl,start_ddl,end_l,end_dl,end_ddl,start_s,end_s);
    a0 = coeff(1);
    a1 = coeff(2);
    a2 = coeff(3);
    a3 = coeff(4);
    a4 = coeff(5);
    a5 = coeff(6);
    % 取10个点计算cost
    ds = zeros(10,1);
    l = zeros(10,1);
    dl = zeros(10,1);
    ddl = zeros(10,1);
    dddl = zeros(10,1);
    for i = 1:10
        ds(i) = start_s + (i-1)*sample_s/10;
    end
    l = a0 * ones(10,1) + a1 * ds + a2 * ds.^2 + a3 * ds.^3 + a4 * ds.^4 + a5 * ds.^5;
    dl = a1 * ones(10,1) + 2 * a2 * ds + 3 * a3 * ds.^2 + 4 * a4 * ds.^3 + 5 * a5 * ds.^4;
    ddl = 2 * a2 * ones(10,1) + 6 * a3 * ds + 12 * a4 * ds.^2 + 20 * a5 * ds.^3;
    dddl = 6 * ones(10,1) * a3 + 24 * a4 * ds + 60 * a5 * ds.^2;
    cost_smooth = w_cost_smooth_dl * (dl' * dl) + w_cost_smooth_ddl * (ddl' * ddl) + w_cost_smooth_dddl * (dddl' * dddl);
    cost_ref = w_cost_ref * (l' * l);
    cost_collision = 0;
    for i = 1:length(obs_s_set)
        if isnan(obs_s_set(i))
            break;
        end
        dlon = ones(10,1) * obs_s_set(i) - ds;
        dlat = ones(10,1) * obs_l_set(i) - l;
        %这里做了非常简化的质点模型，认为障碍物就是一个点
        square_d = dlon.^2 + dlat.^2;
        cost_collision_once = CalcObsCost(w_cost_collision,square_d);
        cost_collision = cost_collision + cost_collision_once;
    end
    cost = cost_collision + cost_smooth + cost_ref;
        
end

function obs_cost = CalcObsCost(w_cost_collision,square_d)
%该函数将计算障碍物的距离代价
% 暂定超过4米的cost为0 在4到3米的cost为1000/squard_d,在小于3米的cost为w_cost_collision
  cost = 0;
  for i = 1:length(square_d)
      if (square_d(i) < 16 && square_d(i) > 9) 
          cost = cost + 1000/square_d(i);
      elseif (square_d(i) < 9)
          cost = cost + w_cost_collision;
      end
  end
  obs_cost = cost;

end

function coeff = CalcQuinticCoeffient(start_l,start_dl,start_ddl,end_l,end_dl,end_ddl,start_s,end_s)
    % l = a0 + a1*s + a2*s^2 + a3*s^3 + a4*s^4 + a5*s^5
    % l' = a1 + 2 * a2 * s + 3 * a3 * s^2 + 4 * a4 * s^3 + 5 * a5 * s^4
    % l'' = 2 * a2 + 6 * a3 * s + 12 * a4 * s^2 + 20 * a5 * s^3
    start_s2 = start_s * start_s;
    start_s3 = start_s2 * start_s;
    start_s4 = start_s3 * start_s;
    start_s5 = start_s4 * start_s;
    end_s2 = end_s * end_s;
    end_s3 = end_s2 * end_s;
    end_s4 = end_s3 * end_s;
    end_s5 = end_s4 * end_s;
    A = [1,start_s, start_s2,     start_s3,     start_s4,      start_s5;
         0 1,       2 * start_s,  3 * start_s2, 4 * start_s3,  5 * start_s4;
         0 0,       2,            6 * start_s,  12 * start_s2, 20 * start_s3;
         1,end_s, end_s2,     end_s3,     end_s4,      end_s5;
         0,1,     2 * end_s,  3 * end_s2, 4 * end_s3,  5 * end_s4;
         0,0,     2,          6 * end_s,  12 * end_s2, 20 * end_s3;];
    B = [start_l;
         start_dl;
         start_ddl;
         end_l;
         end_dl;
         end_ddl;];
     coeff = A \ B;
    
end
